simulink model "xspec_xfer2"  (R2021a)
settings: Solver=VariableStepAuto  StartTime=0.0  StopTime=100*NFFT/Fs  RelTol=1e-6
PreLoadFcn:
  | preload_fcn
StartFcn:
  | tic
StopFcn:
  | trun = toc
values from neighbouring files (symbols this model uses):
  BW = 10e3    (= 10000)    [preload_fcn.m]
  Fs = OSR*BW    (= 25600)    [preload_fcn.m]
  H = tf([1 0 (2*pi*1e3)^2],[1 2*pi*1e3 (2*pi*1e3)^2])    [preload_fcn.m]
  mag = squeeze(mag)    [preload_fcn.m]
  NFFT = 1024    [preload_fcn.m]
  OSR = 2.56    [preload_fcn.m]
  p = 1/AvgFac    (= 0.001)    [preload_fcn.m]
  phz = squeeze(phz)    [preload_fcn.m]
undefined symbols (not defined in the file or in its folder): dfilt, magnitude
libraries: dsparch4 x4, dspsrcs4 x3, dspxfrm3 x2, dspobslib x2, dspsigops x2, simulink_extras x1, dspmathops x1
settings Model: SimulationMode=accelerator  NumberOfSteps=8192  Creator=kschutz  LastModifiedBy=kschutz

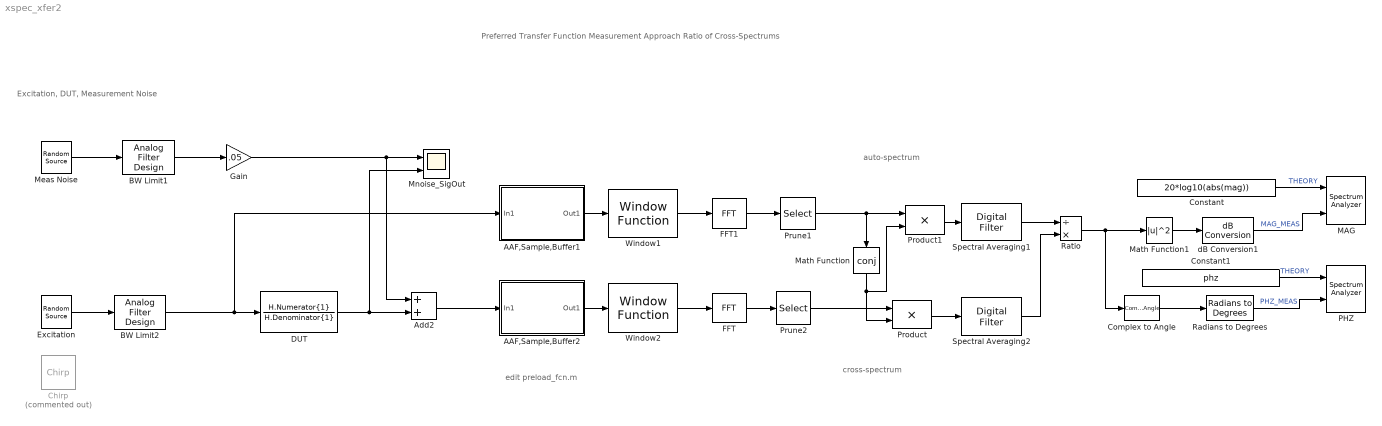
== system xspec_xfer2 ==
  note: auto-spectrum
  note: Excitation, DUT, Measurement Noise
  note: Preferred Transfer Function Measurement Approach
      | Ratio of Cross-Spectrums
  note: edit preload_fcn.m
  note: cross-spectrum
  AAF,Sample,Buffer1 : Subsystem
  AAF,Sample,Buffer2 : Subsystem
  Add2 : Sum
  BW Limit1 : dsparch4/Analog Filter Design  method=Elliptic  filttype=Lowpass  N=8  Wlo=2*pi*BW*10  Whi=80  Rp=2  Rs=80
  BW Limit2 : dsparch4/Analog Filter Design  method=Elliptic  filttype=Lowpass  N=8  Wlo=2*pi*BW  Whi=80  Rp=.5  Rs=80
  Chirp : dspsrcs4/Chirp  Commented=on  sweep=Linear  mode=Unidirectional  f0=0  f1=BW  t1=NFFT/Fs  Tsweep=NFFT/Fs  phase=pi/2  Ts=1/(Fs)  spf=1  datatype=Double  OutputFrames=off
  Complex to Angle : ComplexToMagnitudeAngle  Output=Angle
  Constant : Constant  Value=20*log10(abs(mag))  VectorParams1D=off  SampleTime=(NFFT/OSR)/BW
  Constant1 : Constant  Value=phz  VectorParams1D=off  SampleTime=(NFFT/OSR)/BW
  "DUT  " : TransferFcn  Numerator=H.Numerator{1}  Denominator=H.Denominator{1}
  Excitation : dspsrcs4/Random Source  SrcType=Gaussian  NormMethod=Ziggurat  CltLength=12  MinVal=0  MaxVal=1  MeanVal=0  VarVal=1  RepMode=Specify seed  rawSeed=123  IsInherit=off  SampMode=Discrete  SampTime=1/Fs  SampFrame=1  DataType=Double  OutComplex=Real  OutputFrames=off
  FFT : dspxfrm3/FFT  FFTImplementation=Auto  CompMethod=Table lookup  TableOpt=NEW  TableOptActive=Speed  BitRevOrder=off  Normalize=on  InheritFFTLength=on  FFTLength=64  WrapInput=on  roundingMode=Floor  overflowMode=off  firstCoeffMode=Specify word length  firstCoeffWordLength=16  firstCoeffFracLength=15  firstCoeffDataTypeStr=fixdt(1,16)  firstCoeffLastDataTypeStr=fixdt(1,16)  outputMin=[]  outputMax=[]
  FFT1 : dspxfrm3/FFT  FFTImplementation=Auto  CompMethod=Table lookup  TableOpt=NEW  TableOptActive=Speed  BitRevOrder=off  Normalize=on  InheritFFTLength=on  FFTLength=64  WrapInput=on  roundingMode=Floor  overflowMode=off  firstCoeffMode=Specify word length  firstCoeffWordLength=16  firstCoeffFracLength=15  firstCoeffDataTypeStr=fixdt(1,16)  firstCoeffLastDataTypeStr=fixdt(1,16)  outputMin=[]  outputMax=[]
  Gain : Gain  Gain=.05
  MAG : SpectrumAnalyzer  NumInputPorts=2  IsFrequencyInputMode=1
  Math Function : Math  Operator=conj  SignedPower=on  SaturateOnIntegerOverflow=on
  Math Function1 : Math  Operator=magnitude^2  SignedPower=on  SaturateOnIntegerOverflow=on
  Meas Noise : dspsrcs4/Random Source  SrcType=Gaussian  NormMethod=Ziggurat  CltLength=12  MinVal=0  MaxVal=.01  MeanVal=0  VarVal=1  RepMode=Specify seed  rawSeed=456  IsInherit=off  SampMode=Discrete  SampTime=1/Fs  SampFrame=1  DataType=Double  OutComplex=Real  OutputFrames=off
  Mnoise_SigOut : Scope  NumInputPorts=2
  PHZ : SpectrumAnalyzer  NumInputPorts=2  IsFrequencyInputMode=1
  Product : Product  InputSameDT=on  SaturateOnIntegerOverflow=on  OutDataTypeStr=Inherit: Same as first input
  Product1 : Product  InputSameDT=on  SaturateOnIntegerOverflow=on  OutDataTypeStr=Inherit: Same as first input
  Prune1 : Selector  NumberOfDimensions=2  InputPortWidth=3  IndexOptions=Index vector (dialog),Select all  Indices=[1:NFFT/OSR],1  OutputSizes=1,1
  Prune2 : Selector  NumberOfDimensions=2  InputPortWidth=3  IndexOptions=Index vector (dialog),Select all  Indices=[1:NFFT/OSR],1  OutputSizes=1,1
  Radians to Degrees : simulink_extras/Transformations/Radians to Degrees
  Ratio : Product  Inputs=/*  InputSameDT=on  SaturateOnIntegerOverflow=on  OutDataTypeStr=Inherit: Same as first input
  Spectral Averaging1 : dspobslib/Digital Filter  TypePopup=IIR (poles & zeros)  IIRFiltStruct=Direct form II transposed  AllPoleFiltStruct=Direct form  FIRFiltStruct=Direct form  CoeffSource=Specify via dialog  NumCoeffs=p  DenCoeffs=[1 p-1]  BiQuadCoeffs=[1 0.3 0.4 1 0.1 0.2]  LatticeCoeffs=[0.2 0.4]  denIgnore=on  FiltPerSampPopup=One filter per frame  IC=eps  ICnum=0  ICden=0  roundingMode=Floor  overflowMode=off  ScaleValues=1  scaleValueFracLength=14  stageInFracLength=15  stageOutFracLength=15  FilterSource=Specify via dialog  dfiltObjectName=dfilt.dffir([1 2 1])
      settings: SourceProductBaseCode=DS
  Spectral Averaging2 : dspobslib/Digital Filter  TypePopup=IIR (poles & zeros)  IIRFiltStruct=Direct form II transposed  AllPoleFiltStruct=Direct form  FIRFiltStruct=Direct form  CoeffSource=Specify via dialog  NumCoeffs=p  DenCoeffs=[1 p-1]  BiQuadCoeffs=[1 0.3 0.4 1 0.1 0.2]  LatticeCoeffs=[0.2 0.4]  denIgnore=on  FiltPerSampPopup=One filter per frame  IC=eps  ICnum=0  ICden=0  roundingMode=Floor  overflowMode=off  ScaleValues=1  scaleValueFracLength=14  stageInFracLength=15  stageOutFracLength=15  FilterSource=Specify via dialog  dfiltObjectName=dfilt.dffir([1 2 1])
      settings: SourceProductBaseCode=DS
  Window1 : dspsigops/Window Function  winmode=Apply window to input  wintype=Hann  sampmode=Continuous  samptime=1  N=64  Rs=50  beta=10  winsamp=Periodic  UserWindow=hamming  OptParams=off  UserParams={'symmetric'}  dataType=double  isSigned=on  wordLen=16  udDataType=sfix(16)  fracBitsMode=Best precision  numFracBits=15  roundingMode=Floor  overflowMode=off  numSidelobes=4  sidelobeLevel=-30
      settings: SourceProductBaseCode=DS
  Window2 : dspsigops/Window Function  winmode=Apply window to input  wintype=Hann  sampmode=Continuous  samptime=1  N=64  Rs=50  beta=10  winsamp=Periodic  UserWindow=hamming  OptParams=off  UserParams={'symmetric'}  dataType=double  isSigned=on  wordLen=16  udDataType=sfix(16)  fracBitsMode=Best precision  numFracBits=15  roundingMode=Floor  overflowMode=off  numSidelobes=4  sidelobeLevel=-30
      settings: SourceProductBaseCode=DS
  dB Conversion1 : dspmathops/dB Conversion  dBtype=dB  intype=Power  R=1  fuzz=off
  wires:
  Gain/1 -> Add2/1, Mnoise_SigOut/1
  FFT/1 -> Prune2/1
  Meas Noise/1 -> BW Limit1/1
  AAF,Sample,Buffer1/1(Out1) -> Window1/1
  Window2/1 -> FFT/1
  Window1/1 -> FFT1/1
  FFT1/1 -> Prune1/1
  Complex to Angle/1 -> Radians to Degrees/1
  AAF,Sample,Buffer2/1(Out1) -> Window2/1
  Spectral Averaging2/1 -> Ratio/2
  Spectral Averaging1/1 -> Ratio/1
  "DUT  "/1 -> Mnoise_SigOut/2, Add2/2
  Math Function1/1 -> dB Conversion1/1
  Add2/1 -> AAF,Sample,Buffer2/1(In1)
  Excitation/1 -> BW Limit2/1
  BW Limit2/1 -> AAF,Sample,Buffer1/1(In1), "DUT  "/1
  BW Limit1/1 -> Gain/1
  Ratio/1 -> Complex to Angle/1, Math Function1/1
  Constant/1 -> MAG/1  "THEORY"
  Constant1/1 -> PHZ/1  "THEORY"
  Radians to Degrees/1 -> PHZ/2  "PHZ_MEAS"
  dB Conversion1/1 -> MAG/2  "MAG_MEAS"
  Product1/1 -> Spectral Averaging1/1
  Product/1 -> Spectral Averaging2/1
  Prune1/1 -> Math Function/1, Product1/1
  Prune2/1 -> Product/1
  Math Function/1 -> Product1/2, Product/2

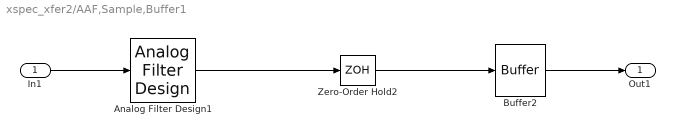
== system xspec_xfer2/AAF,Sample,Buffer1 ==
  In1 : Inport
  Analog Filter Design1 : dsparch4/Analog Filter Design  method=Elliptic  filttype=Lowpass  N=8  Wlo=2*pi*BW  Whi=80  Rp=.5  Rs=80
  Buffer2 : Buffer  N=NFFT  OutputFrames=off
  Zero-Order Hold2 : ZeroOrderHold  SampleTime=1/Fs
  Out1 : Outport
  wires:
  In1/1 -> Analog Filter Design1/1
  Buffer2/1 -> Out1/1
  Analog Filter Design1/1 -> Zero-Order Hold2/1
  Zero-Order Hold2/1 -> Buffer2/1

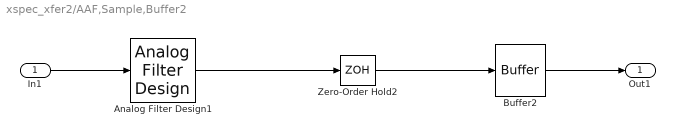
== system xspec_xfer2/AAF,Sample,Buffer2 ==
  In1 : Inport
  Analog Filter Design1 : dsparch4/Analog Filter Design  method=Elliptic  filttype=Lowpass  N=8  Wlo=2*pi*BW  Whi=80  Rp=.5  Rs=80
  Buffer2 : Buffer  N=NFFT  OutputFrames=off
  Zero-Order Hold2 : ZeroOrderHold  SampleTime=1/Fs
  Out1 : Outport
  wires:
  Zero-Order Hold2/1 -> Buffer2/1
  Analog Filter Design1/1 -> Zero-Order Hold2/1
  Buffer2/1 -> Out1/1
  In1/1 -> Analog Filter Design1/1
